simulink model "Simulink_Lab5"  (R2024a)
settings: Solver=VariableStepAuto  StartTime=0.0  StopTime=10.0  RelTol=1e-3
values from neighbouring files (symbols this model uses):
  A = [0,1 ... (first row only)    [Lab5.m]
  ALPHA = inv(-(C-D*K)*inv((A-B*K))*B+D)    [Lab5.m]
  ALPHA1 = inv(-(C-D*K1)*inv((A-B*K1))*B+D)    [Lab5.m]
  B = [0 ... (first row only)    [Lab5.m]
  C = [2, 1]    [Lab5.m]
  K = place(A,B,lambdaK)    [Lab5.m]
  K1 = place(A,B,lambdaK1)    [Lab5.m]
  L = place(A',C',lambdaL)'    [Lab5.m]
  L1 = place(A',C',lambdaL1)'    [Lab5.m]
  L2 = place(A',C',lambdaL2)'    [Lab5.m]
settings Model: Creator=luigi  LastModifiedBy=luigi

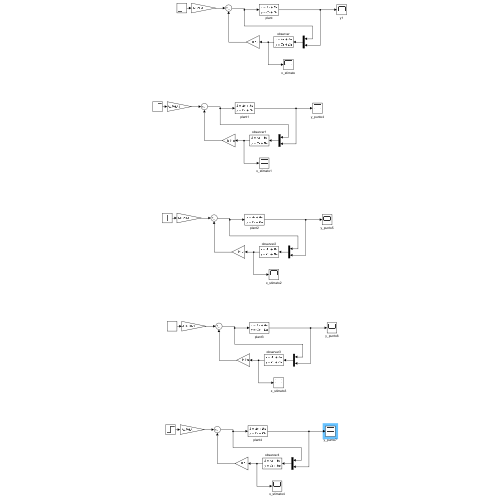
[thumbnail: Simulink's stored preview of the top-level diagram]
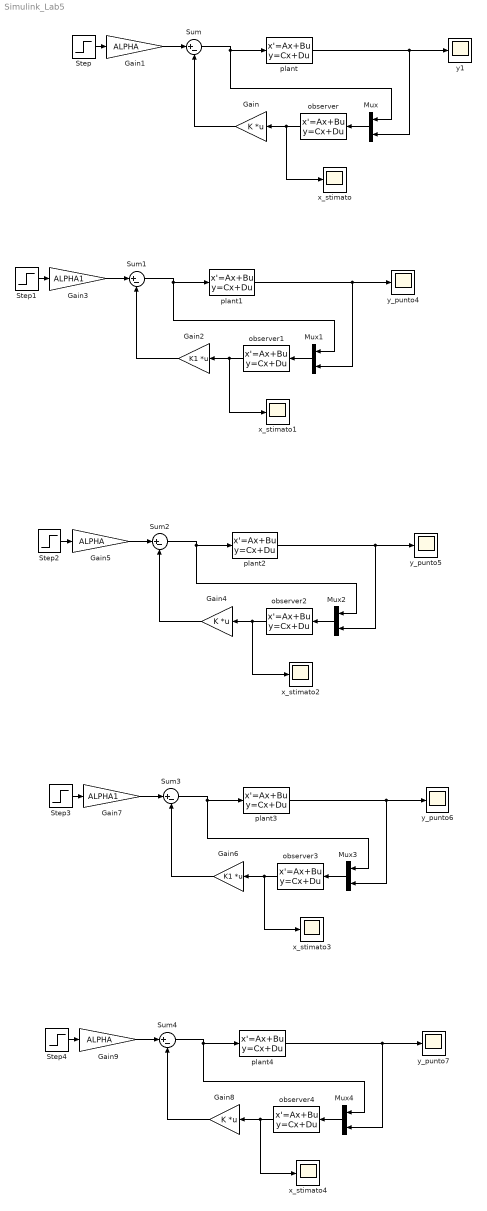
== system Simulink_Lab5 ==
  Gain : Gain  Gain=K  Multiplication=Matrix(K*u)
  Gain1 : Gain  Gain=ALPHA
  Gain2 : Gain  Gain=K1  Multiplication=Matrix(K*u)
  Gain3 : Gain  Gain=ALPHA1
  Gain4 : Gain  Gain=K  Multiplication=Matrix(K*u)
  Gain5 : Gain  Gain=ALPHA
  Gain6 : Gain  Gain=K1  Multiplication=Matrix(K*u)
  Gain7 : Gain  Gain=ALPHA1
  Gain8 : Gain  Gain=K  Multiplication=Matrix(K*u)
  Gain9 : Gain  Gain=ALPHA
  Mux{,1..4} (5 alike) : Mux  Inputs=2
  Step{,1..4} (5 alike) : Step  Time=0  SampleTime=0
  Sum{,1..4} (5 alike) : Sum  Inputs=|+-
  observer : StateSpace  A=A-L*C  B="[B  L]"  C=eye(2)  D=zeros(2,2)  InitialCondition=[0 0]'
  observer1 : StateSpace  A=A-L*C  B="[B  L]"  C=eye(2)  D=zeros(2,2)  InitialCondition=[0 0]'
  observer2 : StateSpace  A=A-L*C  B="[B  L]"  C=eye(2)  D=zeros(2,2)  InitialCondition=[0 0]'
  observer3 : StateSpace  A=A-L1*C  B="[B  L1]"  C=eye(2)  D=zeros(2,2)  InitialCondition=[0 0]'
  observer4 : StateSpace  A=A-L2*C  B="[B  L2]"  C=eye(2)  D=zeros(2,2)  InitialCondition=[0 0]'
  plant{,1,3..4} (4 alike) : StateSpace  A=A  B=B  C=C  D=0  InitialCondition=[0 0]'
  plant2 : StateSpace  A=A  B=B*eps  C=C  D=0  InitialCondition=[0 0]'
  x_stimato{,1..4} (5 alike) : Scope
  y1 : Scope
  y_punto{4..7} (4 alike) : Scope
  wires:
  observer/1 -> x_stimato/1, Gain/1
  Gain/1 -> Sum/2
  Sum/1 -> Mux/1, plant/1
  Gain1/1 -> Sum/1
  Step/1 -> Gain1/1
  Mux/1 -> observer/1
  plant/1 -> y1/1, Mux/2
  Sum1/1 -> Mux1/1, plant1/1
  Gain3/1 -> Sum1/1
  Step1/1 -> Gain3/1
  observer1/1 -> x_stimato1/1, Gain2/1
  Mux1/1 -> observer1/1
  plant1/1 -> y_punto4/1, Mux1/2
  Gain2/1 -> Sum1/2
  Sum2/1 -> Mux2/1, plant2/1
  Step2/1 -> Gain5/1
  plant2/1 -> y_punto5/1, Mux2/2
  observer2/1 -> x_stimato2/1, Gain4/1
  Mux2/1 -> observer2/1
  Gain4/1 -> Sum2/2
  Gain5/1 -> Sum2/1
  Sum3/1 -> Mux3/1, plant3/1
  Gain7/1 -> Sum3/1
  Step3/1 -> Gain7/1
  observer3/1 -> x_stimato3/1, Gain6/1
  Mux3/1 -> observer3/1
  plant3/1 -> y_punto6/1, Mux3/2
  Gain6/1 -> Sum3/2
  Mux4/1 -> observer4/1
  observer4/1 -> x_stimato4/1, Gain8/1
  Step4/1 -> Gain9/1
  Sum4/1 -> Mux4/1, plant4/1
  plant4/1 -> y_punto7/1, Mux4/2
  Gain8/1 -> Sum4/2
  Gain9/1 -> Sum4/1
